simulink model "BDA_DynamicModel_v3"  (R2021b)
settings: Solver=ode23t  StartTime=0.0  StopTime=15  FixedStep=0.000001  MaxStep=1e-5  MinStep=1e-7  RelTol=1e-3
undefined symbols (not defined in the file or in its folder): X, Y, Z
libraries: sm_lib x47, nesl_utility x7
(part 4 of 5)

== matlab function BDA_DynamicModel_v3/PD+g/H ==
  data: q2 input; H output; q3 input; q4 input; q5 input; q6 input
function H = H(q2,q3,q4,q5,q6)
%#codegen

%    This function was generated by the Symbolic Math Toolbox version 9.0.
%    27-Nov-2021 14:09:52

t2 = conj(q2);
t3 = conj(q3);
t4 = conj(q4);
t5 = conj(q5);
t6 = conj(q6);
t7 = cos(q2);
t8 = cos(q4);
t9 = cos(q5);
t10 = cos(q6);
t11 = sin(q2);
t12 = sin(q4);
t13 = sin(q5);
t14 = sin(q6);
t31 = 9.007199254740992e+15;
t15 = cos(t2);
t16 = cos(t4);
t17 = cos(t5);
t18 = cos(t6);
t19 = sin(t2);
t20 = sin(t4);
t21 = sin(t5);
t22 = sin(t6);
t23 = t7.*1.051339e-1;
t24 = t11.*1.051339e-1;
t25 = t9.*5.110348748545983e-1;
t27 = t13.*5.110348748545983e-1;
t30 = t11.*3.235525e-2;
t35 = t7.*3.235525e-2;
t38 = t9.*t12.*8.595599785252598e-1;
t39 = t12.*t13.*8.595599785252598e-1;
t48 = t10.*t13.*4.36041e-5;
t49 = t13.*t14.*4.36041e-5;
t50 = (q3.*t31)./9.007199254740992e+15;
t51 = (t3.*t31)./9.007199254740992e+15;
t56 = q3.*t31.*1.110223024625157e-16i;
t57 = t3.*t31.*1.110223024625157e-16i;
t73 = t10.*1.33637554986e-4;
t74 = t13.*1.33637554986e-4;
t75 = t13.*7.26350557185e-5;
t76 = t14.*7.26350557185e-5;
t77 = t13.*6.1855407534e-5;
t78 = t9.*1.35652563578e-4;
t81 = t9.*t10.*7.26350557185e-5;
t83 = t8.*3.748033925961328e-5;
t84 = t9.*t14.*1.33637554986e-4;
t88 = t13.*t14.*4.35810334311e-7;
t96 = t10.*t13.*8.01825329916e-7;
t110 = t11.*5.850606868813307e-5;
t114 = t7.*1.908064240151374e-5;
t116 = t13.*3.161027044821787e-5;
t117 = t13.*3.711904660916042e-5;
t118 = t9.*6.932319085178867e-5;
t119 = t8.*9.395517395143932e-4;
t120 = t12.*9.395517395143932e-4;
t121 = t9.*3.601891949238275e-7;
t122 = t13.*3.601891949238275e-7;
t123 = t8.*5.316843277159623e-5;
t124 = t12.*1.451749445763287e-4;
t125 = t8.*3.746051216014494e-7;
t126 = t8.*1.166015146360021e-4;
t128 = t13.*6.829345118814501e-5;
t131 = t13.*4.203395243364607e-6;
t132 = t12.*5.427853659906482e-4;
t133 = t9.*7.314371377091851e-7;
t134 = t13.*7.314371377091851e-7;
t135 = t8.*t10.*1.148694938939344e-4;
t136 = t10.*3.387428925624357e-6;
t137 = t9.*t12.*6.243418693357491e-5;
t138 = t8.*t14.*6.243418693357491e-5;
t139 = t9.*t12.*1.148694938939344e-4;
t140 = t9.*t12.*5.316843277159623e-5;
t141 = t10.*1.245668607194124e-6;
t142 = t14.*1.745966317740249e-6;
t143 = t14.*1.245668607194124e-6;
t144 = t12.*t13.*1.166015146360021e-4;
t146 = t8.*t9.*5.427853659906482e-4;
t147 = t8.*t13.*5.427853659906482e-4;
t148 = t9.*t12.*6.058377458913066e-7;
t149 = t12.*t13.*6.058377458913066e-7;
t150 = t8.*1.607033050476913e-7;
t151 = t8.*t9.*3.626595104792852e-4;
t152 = t9.*4.0082304082032e-9;
t153 = t10.*t12.*3.626595104792852e-4;
t154 = t12.*t14.*3.626595104792852e-4;
t155 = t9.*t10.*1.745966317740249e-6;
t158 = t8.*6.892169633636063e-7;
t160 = t9.*t14.*3.387428925624357e-6;
t161 = t9.*t14.*(-1.245668607194124e-6);
t162 = t8.*t10.*t13.*3.626595104792852e-4;
t163 = t8.*t13.*t14.*3.626595104792852e-4;
t166 = t13.*5.918087154269792e-7;
t167 = t9.*2.261852897508832e-6;
t174 = t13.*1.87902861198544e-8;
t198 = t9.*3.73789886133219e-7;
t199 = t13.*3.73789886133219e-7;
t200 = t13.*2.148081562157245e-6;
t202 = t12.*6.769412826196288e-6;
t203 = t8.*2.706536467726674e-6;
t204 = t9.*2.048345525044518e-9;
t205 = t8.*2.289498402241797e-6;
t206 = t12.*3.086744386437578e-6;
t208 = t8.*t13.*6.769412826196288e-6;
t209 = t9.*t12.*3.61307032511966e-6;
t211 = t8.*3.445314443599436e-9;
t212 = t9.*t12.*6.287140903818846e-7;
t213 = t12.*t13.*6.287140903818846e-7;
t214 = t8.*t9.*3.086744386437578e-6;
t215 = t8.*t14.*1.500762770582635e-6;
t216 = t8.*t10.*1.070726881249372e-6;
t217 = t8.*t9.*6.668858699921061e-6;
t218 = t8.*t9.*3.624676635982417e-6;
t219 = t8.*t14.*1.070726881249372e-6;
t220 = t10.*t12.*6.668858699921061e-6;
t221 = t12.*6.078899754658124e-9;
t222 = t12.*t14.*3.624676635982417e-6;
t223 = t8.*t10.*2.911698334565516e-6;
t224 = t12.*3.10211731732776e-5;
t225 = t8.*9.392818914088469e-10;
t226 = t12.*9.392818914088469e-10;
t227 = t8.*t9.*3.517249171619401e-8;
t228 = t12.*t13.*3.445314443599436e-9;
t229 = t8.*t13.*3.517249171619401e-8;
t230 = t8.*t10.*t13.*3.624676635982417e-6;
t231 = t8.*t13.*t14.*6.668858699921061e-6;
t234 = t13.*3.024348928260869e-7;
t235 = t9.*1.155885712417937e-6;
t237 = t12.*t13.*1.944198228009988e-6;
t239 = t9.*t12.*5.086950867234759e-7;
t240 = t13.*9.602491515741889e-9;
t251 = t8.*1.615137793366553e-8;
t262 = t9.*t12.*1.615137793366553e-8;
t263 = t8.*2.84449372366336e-5;
t26 = -t24;
t28 = t15.*1.051339e-1;
t29 = t19.*1.051339e-1;
t32 = t17.*5.110348748545983e-1;
t34 = t21.*5.110348748545983e-1;
t36 = t15.*3.235525e-2;
t37 = t19.*3.235525e-2;
t40 = -t39;
t41 = t16.*5.157359871151559e-3;
t42 = t16.*t18.*8.595599785252598e-1;
t43 = t17.*t20.*8.595599785252598e-1;
t44 = t16.*t22.*8.595599785252598e-1;
t45 = t20.*t21.*8.595599785252598e-1;
t52 = cos(t50);
t53 = sin(t50);
t54 = cos(t51);
t55 = sin(t51);
t58 = exp(t56);
t59 = -t56;
t60 = -t57;
t64 = exp(t57);
t79 = t23+t30;
t80 = -t77;
t85 = t18.*t20.*4.990257941055339e-2;
t86 = t20.*t22.*4.990257941055339e-2;
t89 = t16.*t17.*4.990257941055339e-2;
t90 = -t84;
t92 = t27+t38;
t94 = t16.*t18.*t21.*4.990257941055339e-2;
t95 = t16.*t21.*t22.*4.990257941055339e-2;
t127 = -t118;
t129 = -t121;
t130 = -t122;
t145 = -t134;
t156 = t9.*t141;
t157 = t9.*t143;
t159 = -t148;
t164 = -t160;
t165 = -t162;
t168 = -t166;
t169 = t49+t75;
t171 = t48+t74;
t201 = -t198;
t207 = -t203;
t210 = -t204;
t232 = -t229;
t233 = -t230;
t236 = -t235;
t245 = -t240;
t258 = -t251;
t265 = -t262;
t308 = t73+t76+4.36041e-5;
t328 = t119-8.631097478604537e-5;
t329 = t120+9.554306323645785e-8;
t332 = t124+t150;
t361 = t155+t161;
t382 = t152+t174;
t442 = t88+t96+t131;
t461 = t141+t142+4.35810334311e-7;
t476 = t136+t143+8.01825329916e-7;
t546 = t224+t225+2.208156882018249e-9;
t550 = t226+t263-3.390351827752591e-7;
t33 = -t29;
t46 = -t44;
t47 = -t45;
t61 = 1.0./t58;
t62 = t8.*t52;
t63 = t12.*t52;
t65 = exp(t60);
t66 = t16.*t54;
t67 = t20.*t54;
t68 = t58-1.0;
t82 = t26+t35;
t87 = t28+t37;
t93 = t25+t40;
t97 = -t94;
t98 = t34+t43;
t104 = t52.*1.273194e-2;
t105 = t54.*1.273194e-2;
t170 = t41+t89;
t172 = t10.*t92.*4.36041e-5;
t173 = t14.*t92.*4.36041e-5;
t176 = t52.*3.42298471896e-5;
t178 = t52.*3.07913148585e-5;
t179 = t58.*3.694216783411725e-1;
t180 = t58.*1.305783216588275e-1;
t182 = t52.*3.679077402936e-4;
t183 = t64.*1.305783216588275e-1;
t184 = t64.*3.694216783411725e-1;
t238 = t78+t80;
t241 = t8.*t31.*t53.*5.673626844500105e-17;
t242 = t12.*t31.*t53.*5.673626844500105e-17;
t243 = t9.*t31.*t53.*9.543032792050485e-17;
t244 = t13.*t31.*t53.*9.543032792050485e-17;
t247 = t14.*t92.*4.35810334311e-7;
t252 = t81+t90;
t254 = t16.*t31.*t55.*5.673626844500105e-17;
t255 = t20.*t31.*t55.*5.673626844500105e-17;
t256 = t17.*t31.*t55.*9.543032792050485e-17;
t257 = t21.*t31.*t55.*9.543032792050485e-17;
t261 = t10.*t92.*8.01825329916e-7;
t264 = t16.*t31.*t55.*3.404176106700063e-19;
t266 = t58.*3.215186923359161e-3;
t268 = t58.*1.345257168956303e-2;
t269 = t64.*3.215186923359161e-3;
t270 = t64.*1.345257168956303e-2;
t271 = t52.*8.550795305149304e-7;
t275 = t52.*2.150354518622839e-6;
t283 = t52.*2.380363079699592e-9;
t294 = t31.*t53.*4.87211480085e-18;
t295 = t31.*t55.*4.87211480085e-18;
t298 = t8.*t31.*t53.*2.479366200131245e-18;
t299 = t8.*t31.*t53.*7.351481000981246e-18;
t300 = t12.*t31.*t53.*9.810473427588925e-18;
t301 = t12.*t31.*t53.*4.938358626738924e-18;
t306 = t16.*t31.*t55.*2.479366200131245e-18;
t307 = t20.*t31.*t55.*2.479366200131245e-18;
t313 = t20.*t31.*t55.*7.351481000981246e-18;
t314 = t20.*t31.*t55.*4.938358626738924e-18;
t315 = t8.*t31.*t53.*2.47393392290267e-21;
t316 = t16.*t31.*t55.*7.351481000981246e-18;
t317 = t20.*t31.*t55.*9.810473427588925e-18;
t320 = t58.*1.073174736839591e-5;
t321 = t58.*4.490239736257417e-5;
t324 = t58.*3.887314306731568e-4;
t330 = t31.*t53.*2.127584079327986e-20;
t334 = t31.*t53.*1.611765660673211e-20;
t335 = t13.*t31.*t53.*6.931587185740596e-21;
t336 = t8.*t31.*t53.*7.696420262413979e-21;
t337 = t8.*t31.*t53.*3.509445006623964e-21;
t338 = t9.*t31.*t53.*1.294536862550567e-20;
t339 = t12.*t31.*t53.*5.371403294717661e-20;
t340 = t8.*t31.*t53.*2.472625211857455e-23;
t343 = t13.*t31.*t53.*1.275307569480848e-20;
t345 = t12.*t31.*t53.*9.582443148530891e-21;
t346 = t13.*t31.*t53.*5.902881824626087e-21;
t349 = t9.*t31.*t53.*6.726150146755334e-23;
t350 = t13.*t31.*t53.*6.726150146755334e-23;
t351 = t31.*t53.*1.78416509397307e-23;
t352 = t8.*t31.*t53.*2.503226128461205e-19;
t353 = t12.*t31.*t53.*2.503226128461205e-19;
t354 = t8.*t31.*t53.*1.095358398302466e-19;
t356 = t12.*t31.*t53.*1.06707538424542e-19;
t357 = t12.*t31.*t53.*1.095358398302466e-19;
t359 = t156+t164;
t364 = t8.*t31.*t53.*4.549257716411571e-23;
t365 = t8.*t31.*t53.*1.060741086483328e-23;
t366 = t133+t168;
t367 = t145+t167;
t371 = t31.*t53.*t79.*5.673626844500105e-17;
t378 = t58.*5.594793061269655e-7;
t383 = t58.*2.27206524062708e-6;
t388 = t58.*2.515092356455324e-9;
t392 = t31.*t53.*2.00574854081142e-22;
t393 = t31.*t53.*2.258468230849856e-22;
t394 = t31.*t53.*6.331121467597849e-23;
t396 = t12.*t31.*t53.*1.330815870366286e-21;
t397 = t12.*t31.*t53.*6.699010075846667e-22;
t398 = t9.*t31.*t53.*6.980128590482299e-23;
t399 = t13.*t31.*t53.*6.980128590482299e-23;
t400 = t13.*t31.*t53.*4.011313864537747e-22;
t402 = t12.*t31.*t53.*3.054641854059808e-22;
t403 = t12.*t31.*t53.*6.068308319649908e-22;
t404 = t9.*t31.*t53.*3.825067422357704e-25;
t405 = t8.*t31.*t53.*1.511210377393976e-22;
t409 = t8.*t31.*t53.*4.563917575948183e-22;
t410 = t8.*t31.*t53.*2.274120364292329e-25;
t411 = t31.*t53.*t79.*1.893760189037778e-19;
t412 = t31.*t53.*4.123498135247176e-25;
t415 = t12.*t31.*t53.*3.145845434116526e-21;
t416 = t8.*t31.*t53.*1.279265104253459e-21;
t417 = t21.*t31.*t55.*4.011313864537747e-22;
t419 = t17.*t31.*t55.*3.825067422357704e-25;
t420 = t16.*t31.*t55.*1.511210377393976e-22;
t422 = t12.*t31.*t53.*6.39965864882112e-21;
t423 = t12.*t31.*t53.*7.086968837016952e-25;
t425 = t8.*t31.*t53.*6.199840717099487e-26;
t426 = t12.*t31.*t53.*6.199840717099487e-26;
t432 = t12.*t31.*t53.*1.6195873051144e-24;
t436 = t9.*t31.*t53.*2.158493637172119e-22;
t437 = t13.*t31.*t53.*5.647649977940937e-23;
t441 = t8.*t31.*t53.*1.659646412768137e-22;
t444 = t8.*t31.*t53.*1.066090717454436e-24;
t445 = t31.*t53.*3.909932369564116e-22;
t446 = t13.*t31.*t53.*1.793163166137816e-24;
t447 = t31.*t55.*3.909932369564116e-22;
t448 = t8.*t31.*t53.*2.975797947808626e-21;
t450 = t8.*t31.*t53.*6.22961116251322e-21;
t451 = t21.*t31.*t55.*1.793163166137816e-24;
t459 = t31.*t55.*5.699051429514929e-23;
t464 = t31.*t53.*t79.*1.94207379898051e-21;
t466 = t31.*t53.*t79.*1.746984305586406e-21;
t484 = t31.*t53.*1.428206656218648e-22;
t547 = t123+t129+t146+t149;
t548 = t126+t130+t147+t159;
t549 = t207+t221+2.093791190610393e-6;
t580 = t116+t127+t132+t140+t144;
t682 = t199+t202+t211+t212+t227+t236+t237;
t683 = t201+t206+t213+t232+t234+t239+t258;
t684 = t205+t208+t210+t214+t228+t245+t265;
t69 = t68.^2;
t70 = t65-1.0;
t72 = t67.*(3.0./5.0e+2);
t91 = t33+t36;
t99 = t32+t47;
t102 = t18.*t98.*(3.0./5.0e+2);
t103 = t22.*t98.*(3.0./5.0e+2);
t106 = t63.*2.228474e-2;
t107 = t62.*6.562549e-2;
t108 = t66.*2.228474e-2;
t109 = t67.*2.228474e-2;
t111 = t66.*6.562549e-2;
t115 = t63.*4.36041e-5;
t181 = t61.*3.694216783411725e-1;
t185 = t61.*1.305783216588275e-1;
t186 = t65.*1.305783216588275e-1;
t187 = t65.*3.694216783411725e-1;
t188 = t62.*1.3117937708872e-3;
t189 = t63.*1.3117937708872e-3;
t190 = t63.*1.35652563578e-4;
t191 = t62.*1.688944904408e-4;
t192 = t63.*6.1855407534e-5;
t193 = t63.*4.35810334311e-7;
t194 = t62.*7.13801892181e-4;
t195 = t63.*1.869599668e-7;
t197 = t63.*8.01825329916e-7;
t246 = t14.*t93.*1.33637554986e-4;
t248 = t10.*t93.*7.26350557185e-5;
t249 = -t242;
t250 = -t243;
t259 = -t255;
t260 = -t256;
t267 = t61.*3.215186923359161e-3;
t272 = t61.*1.345257168956303e-2;
t273 = t65.*3.215186923359161e-3;
t274 = t65.*1.345257168956303e-2;
t276 = t62.*8.902265954562403e-6;
t277 = t63.*4.427198467956924e-6;
t279 = t63.*2.663570267859459e-6;
t280 = t62.*4.059291428568442e-6;
t281 = t63.*4.0082304082032e-9;
t282 = t67.*4.427198467956924e-6;
t285 = t67.*2.663570267859459e-6;
t286 = t62.*4.114486328260564e-5;
t287 = t62.*8.487305697640184e-9;
t288 = t62.*1.092747353151976e-9;
t289 = t63.*1.092747353151976e-9;
t290 = t66.*8.487305697640184e-9;
t292 = t63.*2.925194867859459e-6;
t293 = t63.*1.87902861198544e-8;
t296 = t63.*3.814770659661843e-5;
t302 = t14.*t93.*3.387428925624357e-6;
t303 = t10.*t93.*1.745966317740249e-6;
t304 = t93.*t141;
t305 = t93.*t143;
t309 = -t300;
t310 = -t301;
t312 = t10.*t93.*(-1.245668607194124e-6);
t318 = -t313;
t319 = -t317;
t322 = t61.*1.073174736839591e-5;
t323 = t61.*4.490239736257417e-5;
t325 = t61.*3.887314306731568e-4;
t326 = t63.*2.262452815028836e-6;
t327 = t62.*4.33730920504627e-9;
t331 = t63+t241;
t344 = t67+t254;
t347 = -t338;
t348 = -t339;
t358 = -t345;
t360 = -t353;
t362 = -t356;
t363 = -t357;
t368 = -t365;
t372 = t31.*t53.*t82.*9.543032792050485e-17;
t376 = t31.*t55.*t87.*5.673626844500105e-17;
t380 = t61.*5.594793061269655e-7;
t386 = t61.*2.27206524062708e-6;
t389 = t61.*2.515092356455324e-9;
t395 = -t394;
t401 = -t396;
t406 = -t398;
t407 = -t399;
t413 = -t402;
t414 = -t403;
t418 = -t410;
t421 = -t415;
t424 = t31.*t53.*t82.*3.185302114428987e-19;
t427 = -t422;
t428 = -t423;
t430 = -t425;
t431 = -t426;
t435 = -t432;
t439 = -t436;
t449 = -t448;
t452 = -t450;
t460 = -t459;
t469 = t31.*t53.*t82.*3.266565541972299e-21;
t477 = t31.*t53.*t82.*2.938425274050169e-21;
t581 = t117+t137+t154+t165+t173;
t582 = t128+t139+t153+t163+t172;
t583 = t31.*t55.*t549.*9.543032792050485e-17;
t696 = t200+t209+t220+t222+t231+t233+t247+t261;
t71 = t70.^2;
t100 = t18.*t99;
t101 = t22.*t99;
t112 = -t108;
t113 = -t111;
t196 = -t195;
t253 = -t248;
t278 = -t276;
t284 = -t281;
t291 = -t289;
t297 = -t296;
t311 = -t303;
t333 = t62+t249;
t355 = t66+t259;
t369 = t18.*t344;
t370 = t22.*t344;
t375 = -t372;
t377 = t31.*t55.*t91.*9.543032792050485e-17;
t381 = t61.*t69.*7.997968101822611e-3;
t384 = t61.*t69.*5.407940120688672e-3;
t390 = t85+t95+t102;
t391 = t86+t97+t103;
t408 = t13.*t331.*4.334075e-2;
t429 = -t424;
t433 = t17.*t344.*4.334075e-2;
t434 = t21.*t344.*4.334075e-2;
t438 = t61.*t69.*2.669585786930656e-5;
t440 = t61.*t69.*1.805078477303827e-5;
t443 = t61.*t69.*1.56270217221073e-4;
t453 = t61.*t69.*t79.*2.196325630278387e-1;
t454 = t61.*t69.*t82.*2.196325630278387e-1;
t462 = t9.*t331.*4.71413003675e-4;
t463 = t13.*t331.*4.71413003675e-4;
t465 = t73.*t331;
t467 = t9.*t331.*3.149723995125e-4;
t468 = t76.*t331;
t472 = t14.*t331.*4.35810334311e-7;
t475 = -t469;
t480 = -t477;
t481 = t10.*t331.*8.01825329916e-7;
t483 = t61.*t69.*4.313809179931398e-7;
t485 = t61.*t69.*9.133712910180717e-7;
t486 = t61.*t69.*1.011068305420342e-9;
t487 = t61.*t69.*t79.*7.330961578512107e-4;
t488 = t61.*t69.*t82.*7.330961578512107e-4;
t489 = t61.*t69.*t79.*6.346599179580158e-3;
t491 = t9.*t331.*3.148057791131579e-6;
t492 = t13.*t331.*5.879283844893203e-6;
t493 = t9.*t331.*2.68085975407921e-6;
t494 = t9.*t331.*5.791951861259479e-6;
t495 = t136.*t331;
t496 = t9.*t331.*4.57069415115421e-6;
t498 = t141.*t331;
t499 = t142.*t331;
t500 = t143.*t331;
t502 = t9.*t331.*3.054756263814e-8;
t504 = t13.*t331.*3.054756263814e-8;
t509 = t21.*t344.*5.879283844893203e-6;
t510 = t17.*t344.*2.68085975407921e-6;
t512 = t179+t181+2.61156643317655e-1;
t513 = t180+t185+7.38843356682345e-1;
t518 = t183+t186+7.38843356682345e-1;
t519 = t184+t187+2.61156643317655e-1;
t521 = t61.*t69.*t79.*7.517989070303108e-6;
t523 = t61.*t69.*t82.*6.762775401369527e-6;
H = ft_1({t10,t100,t101,t104,t105,t106,t107,t108,t109,t11,t110,t111,t112,t113,t114,t115,t12,t122,t125,t126,t13,t133,t134,t135,t138,t14,t141,t143,t147,t148,t15,t151,t158,t16,t169,t17,t170,t171,t176,t178,t18,t182,t188,t189,t19,t190,t191,t192,t193,t194,t196,t197,t20,t204,t208,t21,t215,t216,t217,t218,t219,t22,t223,t228,t240,t243,t244,t246,t250,t252,t253,t256,t257,t260,t262,t264,t266,t267,t268,t269,t270,t271,t272,t273,t274,t275,t276,t277,t278,t279,t280,t281,t282,t283,t284,t285,t286,t287,t288,t290,t291,t292,t293,t294,t295,t297,t298,t299,t302,t305,t306,t307,t308,t309,t31,t310,t311,t312,t314,t315,t316,t318,t319,t320,t321,t322,t323,t324,t325,t326,t327,t328,t329,t330,t332,t333,t334,t335,t336,t337,t340,t343,t344,t346,t347,t348,t349,t350,t351,t352,t354,t355,t358,t359,t360,t361,t362,t363,t364,t366,t367,t368,t369,t370,t371,t375,t376,t377,t378,t380,t381,t382,t383,t384,t386,t388,t389,t390,t391,t392,t393,t395,t396,t397,t399,t400,t401,t404,t405,t406,t407,t408,t409,t410,t411,t412,t413,t414,t416,t417,t418,t419,t42,t420,t421,t427,t428,t429,t430,t431,t433,t434,t435,t436,t437,t438,t439,t44,t440,t441,t442,t443,t444,t445,t446,t447,t449,t451,t452,t453,t454,t46,t460,t461,t462,t463,t464,t465,t466,t467,t468,t472,t475,t476,t480,t481,t483,t484,t485,t486,t487,t488,t489,t491,t492,t493,t494,t495,t496,t498,t499,t500,t502,t504,t509,t510,t512,t513,t518,t519,t521,t523,t53,t54,t546,t547,t549,t55,t550,t580,t581,t582,t583,t61,t64,t682,t683,t684,t69,t696,t7,t71,t72,t73,t74,t75,t76,t77,t78,t79,t8,t82,t83,t87,t89,t9,t91,t93,t98,t99});
end
function H = ft_1(ct)
t10 = ct{1};
t100 = ct{2};
t101 = ct{3};
t104 = ct{4};
t105 = ct{5};
t106 = ct{6};
t107 = ct{7};
t108 = ct{8};
t109 = ct{9};
t11 = ct{10};
t110 = ct{11};
t111 = ct{12};
t112 = ct{13};
t113 = ct{14};
t114 = ct{15};
t115 = ct{16};
t12 = ct{17};
t122 = ct{18};
t125 = ct{19};
t126 = ct{20};
t13 = ct{21};
t133 = ct{22};
t134 = ct{23};
t135 = ct{24};
t138 = ct{25};
t14 = ct{26};
t141 = ct{27};
t143 = ct{28};
t147 = ct{29};
t148 = ct{30};
t15 = ct{31};
t151 = ct{32};
t158 = ct{33};
t16 = ct{34};
t169 = ct{35};
t17 = ct{36};
t170 = ct{37};
t171 = ct{38};
t176 = ct{39};
t178 = ct{40};
t18 = ct{41};
t182 = ct{42};
t188 = ct{43};
t189 = ct{44};
t19 = ct{45};
t190 = ct{46};
t191 = ct{47};
t192 = ct{48};
t193 = ct{49};
t194 = ct{50};
t196 = ct{51};
t197 = ct{52};
t20 = ct{53};
t204 = ct{54};
t208 = ct{55};
t21 = ct{56};
t215 = ct{57};
t216 = ct{58};
t217 = ct{59};
t218 = ct{60};
t219 = ct{61};
t22 = ct{62};
t223 = ct{63};
t228 = ct{64};
t240 = ct{65};
t243 = ct{66};
t244 = ct{67};
t246 = ct{68};
t250 = ct{69};
t252 = ct{70};
t253 = ct{71};
t256 = ct{72};
t257 = ct{73};
t260 = ct{74};
t262 = ct{75};
t264 = ct{76};
t266 = ct{77};
t267 = ct{78};
t268 = ct{79};
t269 = ct{80};
t270 = ct{81};
t271 = ct{82};
t272 = ct{83};
t273 = ct{84};
t274 = ct{85};
t275 = ct{86};
t276 = ct{87};
t277 = ct{88};
t278 = ct{89};
t279 = ct{90};
t280 = ct{91};
t281 = ct{92};
t282 = ct{93};
t283 = ct{94};
t284 = ct{95};
t285 = ct{96};
t286 = ct{97};
t287 = ct{98};
t288 = ct{99};
t290 = ct{100};
t291 = ct{101};
t292 = ct{102};
t293 = ct{103};
t294 = ct{104};
t295 = ct{105};
t297 = ct{106};
t298 = ct{107};
t299 = ct{108};
t302 = ct{109};
t305 = ct{110};
t306 = ct{111};
t307 = ct{112};
t308 = ct{113};
t309 = ct{114};
t31 = ct{115};
t310 = ct{116};
t311 = ct{117};
t312 = ct{118};
t314 = ct{119};
t315 = ct{120};
t316 = ct{121};
t318 = ct{122};
t319 = ct{123};
t320 = ct{124};
t321 = ct{125};
t322 = ct{126};
t323 = ct{127};
t324 = ct{128};
t325 = ct{129};
t326 = ct{130};
t327 = ct{131};
t328 = ct{132};
t329 = ct{133};
t330 = ct{134};
t332 = ct{135};
t333 = ct{136};
t334 = ct{137};
t335 = ct{138};
t336 = ct{139};
t337 = ct{140};
t340 = ct{141};
t343 = ct{142};
t344 = ct{143};
t346 = ct{144};
t347 = ct{145};
t348 = ct{146};
t349 = ct{147};
t350 = ct{148};
t351 = ct{149};
t352 = ct{150};
t354 = ct{151};
t355 = ct{152};
t358 = ct{153};
t359 = ct{154};
t360 = ct{155};
t361 = ct{156};
t362 = ct{157};
t363 = ct{158};
t364 = ct{159};
t366 = ct{160};
t367 = ct{161};
t368 = ct{162};
t369 = ct{163};
t370 = ct{164};
t371 = ct{165};
t375 = ct{166};
t376 = ct{167};
t377 = ct{168};
t378 = ct{169};
t380 = ct{170};
t381 = ct{171};
t382 = ct{172};
t383 = ct{173};
t384 = ct{174};
t386 = ct{175};
t388 = ct{176};
t389 = ct{177};
t390 = ct{178};
t391 = ct{179};
t392 = ct{180};
t393 = ct{181};
t395 = ct{182};
t396 = ct{183};
t397 = ct{184};
t399 = ct{185};
t400 = ct{186};
t401 = ct{187};
t404 = ct{188};
t405 = ct{189};
t406 = ct{190};
t407 = ct{191};
t408 = ct{192};
t409 = ct{193};
t410 = ct{194};
t411 = ct{195};
t412 = ct{196};
t413 = ct{197};
t414 = ct{198};
t416 = ct{199};
t417 = ct{200};
t418 = ct{201};
t419 = ct{202};
t42 = ct{203};
t420 = ct{204};
t421 = ct{205};
t427 = ct{206};
t428 = ct{207};
t429 = ct{208};
t430 = ct{209};
t431 = ct{210};
t433 = ct{211};
t434 = ct{212};
t435 = ct{213};
t436 = ct{214};
t437 = ct{215};
t438 = ct{216};
t439 = ct{217};
t44 = ct{218};
t440 = ct{219};
t441 = ct{220};
t442 = ct{221};
t443 = ct{222};
t444 = ct{223};
t445 = ct{224};
t446 = ct{225};
t447 = ct{226};
t449 = ct{227};
t451 = ct{228};
t452 = ct{229};
t453 = ct{230};
t454 = ct{231};
t46 = ct{232};
t460 = ct{233};
t461 = ct{234};
t462 = ct{235};
t463 = ct{236};
t464 = ct{237};
t465 = ct{238};
t466 = ct{239};
t467 = ct{240};
t468 = ct{241};
t472 = ct{242};
t475 = ct{243};
t476 = ct{244};
t480 = ct{245};
t481 = ct{246};
t483 = ct{247};
t484 = ct{248};
t485 = ct{249};
t486 = ct{250};
t487 = ct{251};
t488 = ct{252};
t489 = ct{253};
t491 = ct{254};
t492 = ct{255};
t493 = ct{256};
t494 = ct{257};
t495 = ct{258};
t496 = ct{259};
t498 = ct{260};
t499 = ct{261};
t500 = ct{262};
t502 = ct{263};
t504 = ct{264};
t509 = ct{265};
t510 = ct{266};
t512 = ct{267};
t513 = ct{268};
t518 = ct{269};
t519 = ct{270};
t521 = ct{271};
t523 = ct{272};
t53 = ct{273};
t54 = ct{274};
t546 = ct{275};
t547 = ct{276};
t549 = ct{277};
t55 = ct{278};
t550 = ct{279};
t580 = ct{280};
t581 = ct{281};
t582 = ct{282};
t583 = ct{283};
t61 = ct{284};
t64 = ct{285};
t682 = ct{286};
t683 = ct{287};
t684 = ct{288};
t69 = ct{289};
t696 = ct{290};
t7 = ct{291};
t71 = ct{292};
t72 = ct{293};
t73 = ct{294};
t74 = ct{295};
t75 = ct{296};
t76 = ct{297};
t77 = ct{298};
t78 = ct{299};
t79 = ct{300};
t8 = ct{301};
t82 = ct{302};
t83 = ct{303};
t87 = ct{304};
t89 = ct{305};
t9 = ct{306};
t91 = ct{307};
t93 = ct{308};
t98 = ct{309};
t99 = ct{310};
t525 = t61.*t69.*t79.*3.70947298167937e-5;
t527 = t61.*t69.*t79.*4.106249669188362e-8;
t563 = t344.*t382;
t599 = t344.*t550;
t664 = t158+t217+t219+t223+t302+t312;
t697 = t344.*t684;
t175 = t42+t101;
t177 = t46+t100;
t341 = t9.*t333;
t342 = t13.*t333;
t373 = t17.*t355;
t374 = t21.*t355;
t379 = -t377;
t385 = t64.*t71.*7.997968101822611e-3;
t387 = t64.*t71.*5.407940120688672e-3;
t455 = -t454;
t456 = t64.*t71.*t87.*2.196325630278387e-1;
t457 = t64.*t71.*t91.*2.196325630278387e-1;
t490 = -t488;
t501 = t133.*t333;
t503 = t134.*t333;
t506 = -t502;
t524 = -t523;
t538 = t79.*t513;
t539 = t82.*t512;
t541 = t87.*t518;
t542 = t91.*t519;
t590 = t294+t371+t375;
t598 = t355.*t546;
t600 = t266+t267+t381+1.819229615328168e-2;
t601 = -t599;
t624 = t83+t135+t138+t151+t246+t253;
t627 = t330+t411+t429;
t635 = t104+t268+t272+t384+9.510076620873934e-3;
t653 = t393+t464+t475;
t656 = t392+t466+t480;
t661 = t125+t215+t216+t218+t305+t311;
t662 = t178+t320+t322+t438+6.072279186930818e-5;
t663 = t176+t321+t323+t440+3.174301904745164e-5;
t694 = t271+t378+t380+t483+8.856931883486768e-7;
t698 = -t697;
t748 = t182+t191+t196+t324+t325+t358+t368+t443+2.748073584704864e-4;
t458 = -t457;
t470 = t342.*1.35652563578e-4;
t471 = t341.*1.33637554986e-4;
t473 = t341.*7.26350557185e-5;
t474 = t341.*6.1855407534e-5;
t478 = t341.*7.0482312e-7;
t479 = t342.*7.0482312e-7;
t497 = t341.*4.203395243364607e-6;
t505 = t341.*(-7.314371377091851e-7);
t507 = t342.*4.0082304082032e-9;
t511 = t373.*4.203395243364607e-6;
t514 = t374.*4.0082304082032e-9;
t515 = t341.*5.918087154269792e-7;
t516 = t342.*2.261852897508832e-6;
t522 = t341.*1.87902861198544e-8;
t526 = t373.*1.87902861198544e-8;
t528 = t244+t341;
t529 = t250+t342;
t530 = t257+t373;
t531 = t260+t374;
t532 = -t18.*(t256-t374);
t533 = -t22.*(t256-t374);
t534 = t18.*(t256-t374);
t540 = -t539;
t543 = -t542;
t551 = t538.*3.33783e-3;
t552 = t539.*3.33783e-3;
t553 = t539.*2.889644e-2;
t556 = t14.*(t243-t342).*(-1.33637554986e-4);
t558 = t10.*(t243-t342).*(-7.26350557185e-5);
t559 = t10.*(t243-t342).*(-4.35810334311e-7);
t560 = t10.*(t243-t342).*7.26350557185e-5;
t561 = t10.*(t243-t342).*4.35810334311e-7;
t564 = t14.*(t243-t342).*(-8.01825329916e-7);
t567 = t539.*3.42298471896e-5;
t568 = t538.*3.07913148585e-5;
t570 = t539.*1.688944904408e-4;
t572 = t539.*1.869599668e-7;
t574 = t14.*(t243-t342).*(-3.387428925624357e-6);
t575 = t10.*(t243-t342).*(-1.745966317740249e-6);
t576 = -t141.*(t243-t342);
t577 = -t143.*(t243-t342);
t578 = t10.*(t243-t342).*1.745966317740249e-6;
t579 = t10.*(t243-t342).*1.245668607194124e-6;
t585 = -t367.*(t256-t374);
t587 = t367.*(t256-t374);
t591 = t8.*t590;
t592 = t12.*t590;
t594 = t295+t376+t379;
t602 = t8.*t600;
t603 = t12.*t600;
t604 = t269+t273+t385+1.819229615328168e-2;
t605 = t270+t274+t387+9.510076620873934e-3;
t636 = t9.*t635;
t641 = t13.*t635.*7.26735e-3;
t643 = t13.*t635.*1.08769e-2;
t646 = t75.*t635;
t647 = t77.*t635;
t648 = t78.*t635;
t649 = t74.*t635;
t650 = t13.*t635.*(-7.26350557185e-5);
t651 = t13.*t635.*(-6.1855407534e-5);
t652 = t13.*t635.*(-1.33637554986e-4);
t655 = t13.*t635.*7.0482312e-7;
t675 = t31.*t55.*t653.*9.543032792050485e-17;
t676 = t31.*t55.*t656.*5.673626844500105e-17;
t695 = t54.*t694;
t701 = t455+t538+t600;
t712 = -t682.*(t256-t374);
t482 = -t479;
t508 = -t507;
t517 = -t514;
t520 = -t516;
t535 = t18.*t530.*(3.0./5.0e+2);
t536 = t22.*t530.*(3.0./5.0e+2);
t544 = t10.*t528.*4.36041e-5;
t545 = t14.*t528.*4.36041e-5;
t554 = -t552;
t555 = -t553;
t557 = t14.*t528.*4.35810334311e-7;
t562 = t10.*t528.*8.01825329916e-7;
t565 = t22.*t530.*4.35810334311e-7;
t566 = t18.*t530.*8.01825329916e-7;
t569 = -t567;
t571 = -t570;
t573 = -t572;
t584 = t366.*t530;
t588 = t369+t533;
t589 = t370+t534;
t593 = -t592;
t595 = t16.*t594;
t596 = t20.*t594;
t597 = t442.*t530;
t606 = t16.*t604;
t607 = t20.*t604;
t608 = t591.*2.889644e-2;
t609 = t592.*2.889644e-2;
t611 = t592.*1.08769e-2;
t613 = t602.*2.889644e-2;
t614 = t603.*2.889644e-2;
t615 = t602.*1.08769e-2;
t616 = t591.*1.688944904408e-4;
t617 = t592.*6.1855407534e-5;
t618 = t591.*6.678441185616e-4;
t619 = t592.*6.678441185616e-4;
t620 = t592.*1.35652563578e-4;
t625 = t592.*1.869599668e-7;
t628 = t603.*1.688944904408e-4;
t629 = t602.*6.1855407534e-5;
t630 = t602.*6.678441185616e-4;
t631 = t603.*6.678441185616e-4;
t632 = t602.*1.35652563578e-4;
t634 = t602.*1.869599668e-7;
t637 = t105+t605;
t642 = t636.*1.08769e-2;
t644 = -t641;
t645 = -t643;
t654 = t636.*7.0482312e-7;
t665 = t106+t299+t603;
t666 = t107+t309+t602;
t702 = t8.*t701;
t703 = t12.*t701;
t704 = t458+t541+t604;
t705 = t456+t543+t605;
t713 = t530.*t683;
t722 = t453+t540+t635;
t747 = t530.*t696;
t749 = t490+t551+t662;
t537 = -t535;
t586 = -t584;
t610 = -t609;
t612 = -t611;
t621 = -t617;
t622 = -t618;
t623 = -t619;
t626 = -t625;
t633 = -t631;
t638 = t17.*t637;
t639 = t21.*t637;
t657 = t359.*t588;
t658 = t361.*t589;
t659 = t461.*t589;
t660 = t476.*t588;
t667 = t13.*t665;
t668 = t109+t316+t607;
t669 = t108+t318+t606;
t670 = t111+t319+t606;
t678 = t9.*t665.*7.26735e-3;
t679 = t9.*t665.*1.08769e-2;
t680 = t10.*t666.*7.26735e-3;
t681 = t14.*t666.*7.26735e-3;
t685 = t9.*t665.*1.33637554986e-4;
t686 = t9.*t665.*7.26350557185e-5;
t687 = t9.*t665.*6.1855407534e-5;
t689 = t73.*t666;
t690 = t76.*t666;
t691 = t9.*t665.*7.0482312e-7;
t699 = t189+t334+t352+t614;
t700 = t188+t351+t360+t613;
t706 = t16.*t704;
t707 = t20.*t704;
t709 = t702.*2.889644e-2;
t710 = t703.*2.889644e-2;
t711 = t702.*1.08769e-2;
t714 = t703.*1.688944904408e-4;
t715 = t702.*6.1855407534e-5;
t716 = t702.*6.678441185616e-4;
t717 = t703.*6.678441185616e-4;
t718 = t702.*1.35652563578e-4;
t721 = t702.*1.869599668e-7;
t723 = t9.*t722;
t724 = t456+t543+t637;
t729 = t13.*t722.*1.08769e-2;
t730 = t13.*t722.*7.26735e-3;
t733 = t78.*t722;
t734 = t74.*t722;
t735 = t75.*t722;
t736 = t77.*t722;
t737 = t13.*t722.*(-1.33637554986e-4);
t738 = t13.*t722.*(-7.26350557185e-5);
t739 = t13.*t722.*(-6.1855407534e-5);
t740 = t13.*t722.*7.0482312e-7;
t743 = t589.*t661;
t745 = t588.*t664;
t750 = t487+t554+t663;
t763 = t194+t346+t347+t362+t470+t474+t615;
t765 = t106+t298+t591+t703;
t767 = t107+t310+t593+t702;
t789 = t489+t555+t748;
t790 = t277+t287+t416+t435+t445+t628+t634;
t793 = t521+t524+t568+t569+t694;
t798 = t275+t286+t291+t383+t386+t412+t427+t430+t485+t630+1.606199544935468e-6;
t640 = -t639;
t671 = t17.*t668;
t672 = t21.*t668;
t673 = t18.*t670;
t674 = t22.*t670;
t677 = t667.*1.08769e-2;
t688 = t667.*1.35652563578e-4;
t692 = t667.*7.0482312e-7;
t693 = -t691;
t708 = -t706;
t719 = -t717;
t720 = -t718;
t725 = t17.*t724;
t726 = t21.*t724;
t728 = t723.*1.08769e-2;
t731 = -t729;
t732 = -t730;
t741 = t723.*7.0482312e-7;
t742 = -t740;
t744 = -t743;
t746 = -t745;
t751 = t408+t636+t667;
t766 = t13.*t765;
t768 = t109+t306+t595+t707;
t773 = -t18.*(t111-t314-t596+t706);
t774 = -t22.*(t111-t314-t596+t706);
t775 = t22.*(t111-t314-t596+t706);
t776 = t9.*t765.*7.26735e-3;
t777 = t9.*t765.*1.08769e-2;
t779 = t10.*t767.*7.26735e-3;
t780 = t14.*t767.*7.26735e-3;
t781 = t9.*t765.*7.26350557185e-5;
t782 = t9.*t765.*6.1855407534e-5;
t784 = t9.*t765.*1.33637554986e-4;
t785 = t9.*t765.*7.0482312e-7;
t787 = t73.*t767;
t788 = t76.*t767;
t791 = t189+t334+t354+t608+t710;
t792 = t188+t351+t363+t610+t709;
t794 = t31.*t55.*t790.*9.543032792050485e-17;
t795 = t54.*t793;
t797 = t192+t337+t349+t462+t482+t645+t679;
t799 = t283+t288+t297+t388+t389+t395+t431+t452+t486+t633+1.778003609304047e-9;
t800 = t355.*t798;
t805 = t194+t346+t347+t348+t470+t474+t612+t711;
t806 = t115+t315+t465+t467+t468+t556+t560+t644+t678;
t820 = t193+t340+t491+t498+t499+t577+t578+t650+t686;
t821 = t197+t364+t494+t495+t500+t574+t579+t652+t685;
t829 = t275+t286+t291+t383+t386+t412+t421+t430+t485+t525+t571+t623+t716+1.606199544935468e-6;
t831 = (t256-t374).*(t278+t281+t396+t407+t410+t436-t501+t502+t520-t632-t655+t691);
t833 = t277+t287+t409+t428+t445+t616+t626+t714+t721;
t727 = -t726;
t752 = t434+t638+t672;
t753 = t433+t640+t671;
t757 = t10.*t751.*7.26735e-3;
t758 = t14.*t751.*7.26735e-3;
t760 = t14.*t751.*1.33637554986e-4;
t761 = t10.*t751.*7.26350557185e-5;
t769 = t112+t307+t596+t708;
t770 = t17.*t768;
t771 = t21.*t768;
t772 = t113+t314+t596+t708;
t778 = t766.*1.08769e-2;
t783 = t766.*1.35652563578e-4;
t786 = t766.*7.0482312e-7;
t796 = t190+t336+t350+t463+t478+t642+t677;
t801 = t344.*t799;
t809 = t408+t723+t766;
t823 = t589.*t820;
t824 = t588.*t821;
t825 = t276+t284+t399+t401+t418+t439+t501+t506+t516+t632+t655+t693;
t827 = t192+t337+t349+t462+t482+t731+t777;
t828 = t280+t293+t406+t414+t437+t444+t503+t504+t515+t629+t654+t692;
t830 = t283+t288+t297+t388+t389+t395+t431+t449+t486+t527+t573+t622+t719+1.778003609304047e-9;
t834 = t355.*t829;
t837 = t31.*t55.*t833.*9.543032792050485e-17;
t838 = t115+t315+t465+t467+t468+t556+t560+t732+t776;
t839 = t279+t404+t405+t446+t492+t493+t508+t522+t648+t651+t687+t688;
t840 = t193+t340+t491+t498+t499+t577+t578+t738+t781;
t841 = t197+t364+t494+t495+t500+t574+t579+t737+t784;
t851 = t278+t281+t397+t407+t410+t436+t502+t505+t520+t620+t720+t742+t785;
t754 = t22.*t752;
t755 = t18.*t752;
t759 = -t758;
t762 = -t760;
t764 = t72+t264+t753;
t802 = -t801;
t807 = t335+t473+t545+t681+t757;
t810 = t10.*t809.*7.26735e-3;
t811 = t14.*t809.*7.26735e-3;
t813 = t434+t725+t771;
t814 = t433+t727+t770;
t817 = t14.*t809.*1.33637554986e-4;
t818 = t10.*t809.*7.26350557185e-5;
t826 = t190+t336+t350+t463+t478+t728+t778;
t832 = t530.*t828;
t835 = t344.*t830;
t842 = t344.*t839;
t845 = t589.*t840;
t846 = t588.*t841;
t852 = t280+t293+t406+t413+t437+t444+t503+t504+t515+t621+t715+t741+t786;
t853 = -t851.*(t256-t374);
t854 = t851.*(t256-t374);
t856 = t279+t404+t405+t446+t492+t493+t508+t522+t733+t739+t782+t783;
t756 = -t754;
t803 = t536+t674+t755;
t808 = t343+t471+t544+t680+t759;
t812 = -t811;
t815 = t18.*t813;
t816 = t22.*t813;
t819 = -t817;
t822 = t72+t264+t814;
t836 = -t835;
t847 = t335+t473+t545+t780+t810;
t849 = t400+t497+t557+t562+t689+t690+t761+t762;
t855 = t530.*t852;
t857 = t344.*t856;
t804 = t535+t673+t756;
t843 = t537+t773+t816;
t844 = t536+t775+t815;
t848 = t343+t471+t544+t779+t812;
t850 = t530.*t849;
t858 = t400+t497+t557+t562+t787+t788+t818+t819;
t859 = t530.*t858;
et1 = t7.*(-6.595899203175001e-4)+t11.*2.143246017993e-3;
et2 = 4.573233567645e-4;
et3 = t110+t114+t675+t676+t795+t834+t836+t837+t845+t846+t854+t855+t857+t859+t848.*(t535-t816+t18.*(t111-t314-t596+t706))+t594.*t627+t704.*t749+t705.*t750+t724.*t789+t768.*t791+t813.*t826+t814.*t827+t822.*t838+t844.*t847-t91.*(et1+et2)+t792.*(t108-t307-t596+t706)+t805.*(t111-t314-t596+t706);
et4 = t87.*(t7.*2.143246017993e-3+t11.*6.595899203175001e-4+3.222314966007e-4);
et5 = 2.531318772537663e-4;
et6 = t326+t327+t484+t591.*8.631097478604537e-5;
et7 = t592.*(-9.554306323645785e-8);
et8 = t702.*9.554306323645785e-8;
et9 = t703.*8.631097478604537e-5-t16.*t791.*1.264860527128474e-2;
et10 = t20.*t792.*1.264860527128474e-2+t20.*t805.*4.990257941055339e-2+t16.*t830.*8.595599785252598e-1;
et11 = t20.*t829.*8.595599785252598e-1-t16.*t856.*8.595599785252598e-1+t98.*t852+t99.*t851+t98.*t858-t170.*t838-t175.*t841+t390.*t848+t391.*t847-t840.*(t44-t100);
et12 = t8.*t31.*t53.*2.332321047271381e-22;
et13 = t12.*t31.*t53.*(-3.621688232723396e-25);
et14 = t31.*t53.*t79.*(-5.091703513734173e-22);
et15 = t31.*t53.*t82.*8.564238525144865e-22;
et16 = t16.*t17.*t827.*(-4.990257941055339e-2)-t16.*t21.*t826.*4.990257941055339e-2;
et17 = t15.*1.908064240151374e-5+t19.*5.850606868813307e-5+t695;
et18 = t794+t800+t802+t823+t824+t831+t832+t842+t850+t808.*(t535-t816+t18.*(t111-t314-t596+t706))+t53.*t55.*2.671802235009627e-6+t330.*t594;
et19 = t662.*t704+t663.*t705+t699.*t768+t724.*t748+t796.*t813+t797.*t814+t806.*t822+t807.*t844+t700.*(t108-t307-t596+t706)+t763.*(t111-t314-t596+t706)+1.896268252195649e-5;
et20 = t695+t794+t800+t802+t823+t824+t831+t832+t842+t850+t53.*t55.*1.108156578290307e-5+t604.*t662+t605.*t663+t668.*t699+t669.*t700+t637.*t748+t670.*t763+t752.*t796;
et21 = t753.*t797+t764.*t806+t803.*t807+t804.*t808+1.896268252195649e-5;
et22 = t326+t327+t484+t602.*9.554306323645785e-8;
et23 = t603.*8.631097478604537e-5-t16.*t699.*1.264860527128474e-2;
et24 = t20.*t700.*1.264860527128474e-2+t20.*t763.*4.990257941055339e-2+t16.*t799.*8.595599785252598e-1;
et25 = t20.*t798.*8.595599785252598e-1-t16.*t839.*8.595599785252598e-1+t98.*t828+t98.*t849-t170.*t806-t175.*t821+t390.*t808+t391.*t807-t820.*(t44-t100)+t99.*(t278+t281+t396+t407+t410+t436-t501+t502+t520-t632-t655+t691);
et26 = t8.*t31.*t53.*6.53749082458021e-22;
et27 = t12.*t31.*t53.*(-8.276655957852335e-25);
et28 = t16.*t17.*t797.*(-4.990257941055339e-2)-t16.*t21.*t796.*4.990257941055339e-2;
et29 = t460+t583+t598+t601+t698+t712+t713+t744+t746+t747+t582.*(t535-t816+t18.*(t111-t314-t596+t706))+t332.*t724-t328.*t768-t547.*t814+t581.*t844-t624.*t822+t813.*(t122-t126-t147+t148)+t329.*(t108-t307-t596+t706)+t580.*(t111-t314-t596+t706);
et30 = t31.*t55.*t87.*(-5.091703513734173e-22);
et31 = t31.*t55.*t91.*8.564238525144865e-22;
et32 = t8.*(-1.383134525074107e-6);
et33 = t12.*3.106529775375363e-9;
et34 = t16.*t328.*1.264860527128474e-2+t20.*t329.*1.264860527128474e-2+t16.*t550.*8.595599785252598e-1;
et35 = t20.*t546.*8.595599785252598e-1+t20.*t580.*4.990257941055339e-2+t89.*t547+t16.*t684.*8.595599785252598e-1+t98.*t683-t99.*t682+t98.*t696+t170.*t624+t175.*t664+t390.*t582+t391.*t581+t661.*(t44-t100);
et36 = t16.*t21.*(t122-t126-t147+t148).*(-4.990257941055339e-2);
et37 = 1.284998062810757e-6;
et38 = t8.*(-2.514380437799477e-6)+t204-t208-t228+t240+t262;
et39 = t8.*t9.*(-5.262701449313289e-6);
et40 = t8.*t10.*(-6.892169633636063e-7);
et41 = t8.*t14.*(-3.746051216014494e-7)+t10.*t93.*4.35810334311e-7;
et42 = t14.*t93.*(-8.01825329916e-7)-t18.*t664-t22.*t661;
et43 = t282+t290+t447+t563+t586+t587+t595.*1.688944904408e-4-t596.*1.869599668e-7+t597+t657+t658;
et44 = t706.*1.869599668e-7+t707.*1.688944904408e-4+t171.*(t535-t816+t18.*(t111-t314-t596+t706));
et45 = t9.*t814.*7.0482312e-7+t13.*t813.*7.0482312e-7+t169.*t844+t252.*t822+(t77-t78).*(t111-t314-t596+t706);
et46 = t16.*t31.*t55.*4.563917575948183e-22;
et47 = t20.*t31.*t55.*(-7.086968837016952e-25);
et48 = t282+t290+t447+t563+t586+t587+t597+t606.*1.869599668e-7+t607.*1.688944904408e-4+t657+t658;
et49 = t9.*t753.*7.0482312e-7+t13.*t752.*7.0482312e-7+t169.*t803+t171.*t804+t252.*t764+t670.*(t77-t78);
et50 = t16.*t31.*t55.*1.279265104253459e-21;
et51 = t20.*t31.*t55.*(-1.6195873051144e-24);
et52 = t16.*(-2.706536467726674e-6);
et53 = t20.*6.078899754658124e-9-t16.*t382.*8.595599785252598e-1-t170.*t252-t98.*t366+t99.*t367-t175.*t359+t98.*t442;
et54 = t169.*t391+t171.*t390+t20.*(t77-t78).*4.990257941055339e-2-t361.*(t44-t100);
et55 = t9.*t16.*t17.*(-3.517249171619401e-8);
et56 = t13.*t16.*t21.*(-3.517249171619401e-8);
et57 = 2.093791190610393e-6;
et58 = t285+t419+t420+t451+t509+t510+t517+t526+t659+t660+t725.*1.35652563578e-4-t726.*6.1855407534e-5;
et59 = t770.*6.1855407534e-5+t771.*1.35652563578e-4+t308.*t822;
et60 = t285+t419+t420+t451+t509+t510+t517+t526+t638.*1.35652563578e-4-t639.*6.1855407534e-5+t659+t660;
et61 = t671.*6.1855407534e-5+t672.*1.35652563578e-4+t308.*t764;
et62 = t16.*(-2.289498402241797e-6);
et63 = t17.*2.048345525044518e-9;
et64 = t21.*9.602491515741889e-9;
et65 = t16.*t17.*(-3.086744386437578e-6);
et66 = t16.*t21.*(-6.769412826196288e-6);
et67 = t17.*t20.*1.615137793366553e-8;
et68 = t20.*t21.*(-3.445314443599436e-9)-t170.*t308-t175.*t476-t461.*(t44-t100);
et69 = t17.*4.0082304082032e-9;
et70 = t21.*1.87902861198544e-8+t17.*t18.*t461-t17.*t22.*t476;
et71 = t10.*8.01825329916e-7+t14.*4.35810334311e-7+t22.*t461+t18.*t476;
et72 = 2.925194867859459e-6;
et73 = t417+t511+t565+t566+t775.*7.26350557185e-5+t815.*7.26350557185e-5;
et74 = t816.*(-1.33637554986e-4)+t18.*(t111-t314-t596+t706).*1.33637554986e-4;
et75 = t417+t511+t565+t566+t673.*1.33637554986e-4+t674.*7.26350557185e-5;
et76 = t754.*(-1.33637554986e-4)+t755.*7.26350557185e-5;
et77 = t21.*2.148081562157245e-6;
et78 = t17.*t20.*3.61307032511966e-6;
et79 = t18.*t20.*6.668858699921061e-6;
et80 = t20.*t22.*3.624676635982417e-6;
et81 = t18.*t98.*8.01825329916e-7+t22.*t98.*4.35810334311e-7;
et82 = t16.*t18.*t21.*(-3.624676635982417e-6);
et83 = t16.*t21.*t22.*6.668858699921061e-6;
et84 = t21.*4.203395243364607e-6+t18.*t21.*8.01825329916e-7;
et85 = t21.*t22.*4.35810334311e-7;
mt1 = [et3+et4+et5,et17+et18+et19,et29+et30+et31,et43+et44+et45+et46+et47,et58+et59,et73+et74,t110+t114+t675+t676+t795+t834+t836+t837+t845+t846+t854+t855+t857+t859+t295.*t627+t604.*t749+t605.*t750+t637.*t789+t668.*t791+t669.*t792+t670.*t805+t752.*t826+t753.*t827+t764.*t838+t803.*t847+t804.*t848+1.896268252195649e-5,et20+et21];
mt2 = [t460+t583+t598+t601+t698+t712+t713+t744+t746+t747+t332.*t637-t328.*t668+t329.*t669+t580.*t670-t547.*t753+t581.*t803+t582.*t804-t624.*t764+t752.*(t122-t126-t147+t148),et48+et49+et50+et51,et60+et61,et75+et76,et6+et7+et8+et9+et10+et11+et12+et13+et14+et15+et16,et22+et23+et24+et25+et26+et27+et28,et32+et33+et34+et35+et36+et37,et52+et53+et54+et55+et56+et57,et62+et63+et64+et65+et66+et67+et68,et77+et78+et79+et80+et81+et82+et83,t833+t17.*t851+t21.*t852+t21.*t858+t17.*t18.*t840-t17.*t22.*t841+t18.*t21.*t848.*(3.0./5.0e+2)+t21.*t22.*t847.*(3.0./5.0e+2)];
mt3 = [t790+t21.*t828+t21.*t849+t17.*(t278+t281+t396+t407+t410+t436-t501+t502+t520-t632-t655+t691)+t18.*t21.*t808.*(3.0./5.0e+2)+t21.*t22.*t807.*(3.0./5.0e+2)+t17.*t18.*t820-t17.*t22.*t821,t549-t17.*t682+t21.*t683+t21.*t696+t18.*t21.*t582.*(3.0./5.0e+2)+t21.*t22.*t581.*(3.0./5.0e+2)-t17.*t18.*t661+t17.*t22.*t664];
mt4 = [t17.*t367-t21.*t366+t21.*t442+t18.*t21.*t171.*(3.0./5.0e+2)+t21.*t22.*t169.*(3.0./5.0e+2)+t17.*t18.*t361-t17.*t22.*t359+4.097159105249182e-6,et69+et70,et84+et85];
mt5 = [t292+t404+t441+t446+t472+t481+t492+t496+t508+t522+t561+t564+t733+t783-t13.*t722.*1.05459507534e-4+t9.*t765.*1.05459507534e-4+t18.*t841+t22.*t840];
mt6 = [t292+t404+t441+t446+t472+t481+t492+t496+t508+t522+t561+t564+t648+t688-t13.*t635.*1.05459507534e-4+t9.*t665.*1.05459507534e-4+t18.*t821+t22.*t820,et38+et39+et40+et41+et42];
mt7 = [t382+t9.*t10.*4.35810334311e-7-t9.*t14.*8.01825329916e-7+t18.*t359+t22.*t361,et71+et72,0.0,t858,t849,t696,t442,0.0];
mt8 = [4.203395243364607e-6];
H = real(reshape([mt1,mt2,mt3,mt4,mt5,mt6,mt7,mt8],6,6));
end

== matlab function BDA_DynamicModel_v3/PD+g/MATLAB Function ==
  data: H input; Kp output; ts input; Kd output
function [Kp, Kd] = ganancias(H,ts)
Kp = zeros(6,1);
Kd = zeros(6,1);

wn = 6/ts;

for i = 1:6
    Kp(i) = H(i,i)*(wn^2);
    Kd(i) = H(i,i)*(2*(wn^2))-0.002;
end

== matlab function BDA_DynamicModel_v3/PD+g/MATLAB Function1 ==
  data: Kp input; tau output; Kd input; e input; dq input; g input
function tau = PD_g(Kp,Kd,e,dq,g)
    tau = Kp.*e - Kd.*dq + g;

== matlab function BDA_DynamicModel_v3/Energy Analysis/MATLAB Function ==
  data: dq input; T output; H input
function T = Kinetic_Energy(dq, H)
T = real((1/2)*transpose(dq)*H*dq);
